simulink model "missile_forDLZ"  (R2018b)
settings: Solver=ode4  StartTime=0.0  StopTime=inf  FixedStep=0.03  RelTol=1e-3
values from neighbouring files (symbols this model uses):
  CD0 = [0.0599 0.0518 0.1235 0.1695 0.1488 0.1438 0.1405 0.133 0.1246 0.1217 0.1217]    [coe.mat]
  CDi = [0 0.131 0.1425 0.1672 0.2444 0.3738 0.6187 1.0569 1.3652 2.4712 2.9851]    [coe.mat]
  CL_idx = [0 0.2 0.4 0.6 0.8 1 1.2 1.4 1.6 2 4]    [coe.mat]
  CLmax = [2.33 2.43 2.82 2.52 2.24 1.98 1.74 1.19 0.78 0.61 0.61]    [coe.mat]
  ma_idx = [0 0.8 1 1.2 1.4 1.6 1.8 2.4 3.5 4 10]    [coe.mat]
undefined symbols (not defined in the file or in its folder): g, GP_switch, halfa_seeker_lock, init_m, init_t, K, mass, motion_style, nn_lim, overload, overload_height, r_seeker_active, S, TGO_max, thrust, thrust_time_idx, turn_omega, turn_omega_height
libraries: simulink_extras x2, aerolibasang x2, sharedutil x1, aerolibatmos2 x1, aerolibconvert2 x1
(part 2 of 2)

== matlab function missile_forDLZ/missile/PNG/MATLAB Function ==
  settings: updateMethod=DISCRETE
  data: r input; h input; TA input; ny_coe output; AO input
function ny_coe = fcn(r, h, TA, AO)
    persistent coe;
    if isempty(coe)
        TA_coe_max = 7; TA_coe_min = 2;
        AO_coe_max = 7; AO_coe_min = 2;
        r_coe_max = 7; r_coe_min = 2;
        h_coe_max = 3; h_coe_min = 2;
        AO_max = 60;%degree
        r_max = 80;  r_min = 20;%km
        h_max = 15; h_mid = 10; h_min = 5;%km
        n_max = 3;%g

        TA_abs = abs(rad2deg(TA));
        AO_abs = abs(rad2deg(AO));
        r = r / 1000.0;
        h = h / 1000.0;

        TA_coe = TA_coe_max - (TA_coe_max-TA_coe_min)/180*TA_abs;
        if AO_abs > AO_max
            AO_coe = AO_coe_max;
        else
            AO_coe = AO_coe_max - (AO_coe_max-AO_coe_min)/AO_max*AO_abs;
        end
        if r > r_max
            r_coe = r_coe_max;
        elseif r < r_min
            r_coe = r_coe_min;
        else
            r_coe = r_coe_max - (r_coe_max-r_coe_min)/(r_max-r_min)*(r_max-r);
        end
        if h >= h_min && h <= h_mid
            h_coe = h_coe_min + (h_coe_max-h_coe_min)/(h_mid-h_min)*(h-h_min);
        elseif h >= h_mid && h <= h_max
            h_coe = h_coe_max - (h_coe_max-h_coe_min)/(h_max-h_mid)*(h-h_mid);
        else
            h_coe = h_coe_min;
        end
        coe = n_max * (TA_coe+AO_coe+r_coe+h_coe) / (TA_coe_max+AO_coe_max+r_coe_max+h_coe_max);
    end
    
    ny_coe = coe;
end
